simulink model "parte3_eje7_SMIB_NoExc"  (R2019b)
settings: Solver=ode45  StartTime=0.0  StopTime=20  RelTol=1e-3  EnableMultiTasking=on
model workspace (MAT data in the model file):
  D = 0
  F = 60
  H = 6.5
  KAe = 200
  T1e = 1
  T1p = 0.648927607606
  T2e = 10
  T2p = 0.216309202535
  T3 = 1.40659340659
  T3p = 0.648927607606
  T4p = 0.216309202535
  Tee = 0.01
  Tre = 0.01
  Twp = 10
  k1 = 2.21807614913
  k2 = 3.1205207777
  k3 = 0.175824175824
  k4 = 4.68078116655
  k5 = -0.130081858844
  k6 = 0.00523421739465
values from neighbouring files (symbols this model uses):
  K1 = Eb*eqo/D*(RT*sin(do)+XTD*cos(do))+Eb*iqo/D*(xq-xpd)*(XTQ*sin(do)-RT*cos(do))    [parte3_eje2_SMIB_Exc_graph.m]
  K2 = Lads/(Lads+Lfd)*(RT/D*eqo+(XTQ*(xq-xpd)/D+1)*iqo)    [parte3_eje2_SMIB_Exc_graph.m]
  K3 = (Lads+Lfd)/Ladu*1/(1+XTQ/D*(xd+xpd))    (= 0.286464655633)    [parte3_eje2_SMIB_Exc_graph.m]
  K4 = Eb/D*(xd-xpd)*(XTQ*sin(do)-RT*cos(do))    [parte3_eje2_SMIB_Exc_graph.m]
  K5 = -(vdo/Et)*xq*Eb*cos(do)/(xe+xq)-(vqo/Et)*xpd*Eb*sin(do)/(xe+xpd)    [parte3_eje2_SMIB_Exc_graph.m]
  K6 = xe*(vqo/Et)/(xe+xpd)    [parte3_eje2_SMIB_Exc_graph.m]
  Kd = 10    [parte3_eje2_SMIB_Exc_graph.m]
  Tr = 0.01    [parte3_eje2_SMIB_Exc_graph.m]    (also in parte3_eje3_EXAC1.m; parte3_eje3_EXAC2.m; parte3_eje5_ESSTB.m = 0.3)
settings Model: Creator=ramos  LastModifiedBy=cjuar
settings DataIOCC: LimitDataPoints=on  SaveFormat=Array  SignalLoggingSaveFormat=ModelDataLogs  ReturnWorkspaceOutputs=off
settings OptimizationCC: ExpressionDepthLimit=2147483647  LifeSpan=inf
settings DebuggingCC: UnderspecifiedInitializationDetection=Classic  MergeDetectMultiDrivingBlocksExec=none  SolverPrmCheckMsg=warning  FcnCallInpInsideContextMsg=warning  StateNameClashWarn=warning  SFUnexpectedBacktrackingDiag=warning  SFNoUnconditionalDefaultTransitionDiag=warning  SFExecutionAtInitializationDiag=none  ArithmeticOperatorsInVariantConditions=warning
settings HardwareCC: ProdBitPerPointer=32  ProdBitPerSizeT=32  ProdBitPerPtrDiffT=32  ProdLargestAtomicFloat=None  ProdIntDivRoundTo=Undefined  ProdEndianess=Unspecified  ProdWordSize=32  ProdHWDeviceType=32-bit Generic
settings ModelReferenceCC: PropagateSignalLabelsOutOfModel=off
settings SFSimCC: SimUseLocalCustomCode=off  CustomCodeUndefinedFunction=UseInterfaceOnly
settings RTWCC: RTWUseLocalCustomCode=off
settings CodeAppCC: StateflowObjectComments=on
settings GRTTargetCC: TargetLangStandard=C89/C90 (ANSI)  GeneratePreprocessorConditionals=Disable all  CombineOutputUpdateFcns=off  GRTInterface=on
settings ConfigComp: CovMetricSettings=dw  CovHtmlReporting=on  CovSaveCumulativeToWorkspaceVar=on  CovSaveSingleToWorkspaceVar=on  CovExternalEMLEnable=off

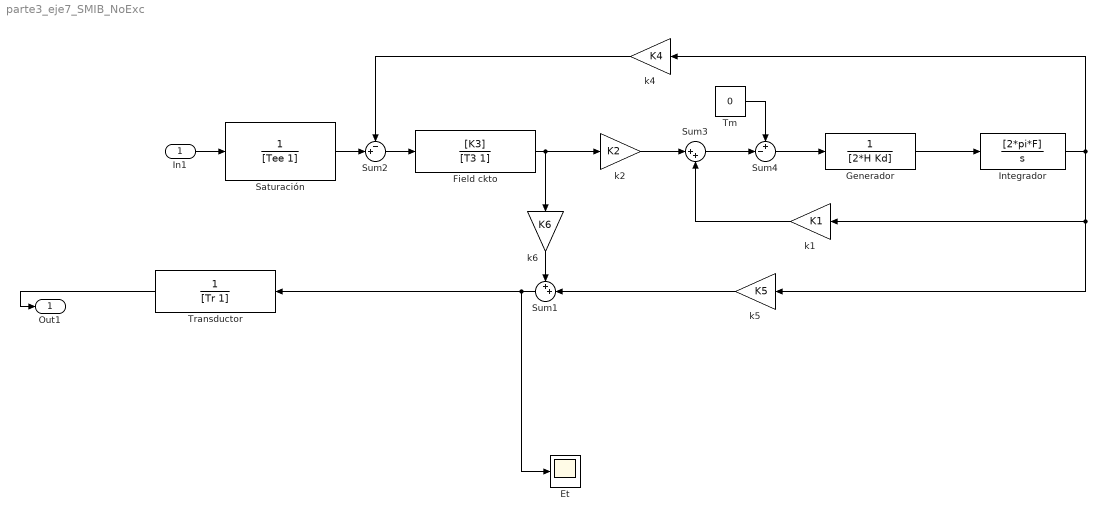
== system parte3_eje7_SMIB_NoExc ==
  In1 : Inport
  Et : Scope
  Field ckto : TransferFcn  Numerator=[K3]  Denominator=[T3 1]
  Generador : TransferFcn  Denominator=[2*H Kd]
  Integrador : TransferFcn  Numerator=[2*pi*F]  Denominator=[1 0]
  Saturación : TransferFcn  Denominator=[Tee 1]
  Sum1 : Sum  Inputs=++|
  Sum2 : Sum  Inputs=-+|
  Sum3 : Sum  Inputs=|++
  Sum4 : Sum  Inputs=+-|
  Tm : Constant  Value=0
  Transductor : TransferFcn  Denominator=[Tr 1]
  k1 : Gain  Gain=K1
  k2 : Gain  Gain=K2
  k4 : Gain  Gain=K4
  k5 : Gain  Gain=K5
  k6 : Gain  Gain=K6
  Out1 : Outport
  wires:
  Field ckto/1 -> k2/1, k6/1
  k6/1 -> Sum1/1
  Sum2/1 -> Field ckto/1
  k4/1 -> Sum2/1
  k5/1 -> Sum1/2
  k2/1 -> Sum3/1
  k1/1 -> Sum3/2
  Sum3/1 -> Sum4/2
  Tm/1 -> Sum4/1
  Sum4/1 -> Generador/1
  Generador/1 -> Integrador/1
  Integrador/1 -> k1/1, k5/1, k4/1
  Sum1/1 -> Et/1, Transductor/1
  In1/1 -> Saturación/1
  Transductor/1 -> Out1/1
  Saturación/1 -> Sum2/2
